simulink subsystem "mode_xxI"  (R2022a)
settings: Solver=VariableStepAuto  StartTime=0.0  StopTime=10.0  RelTol=1e-3
settings Model: Creator=bkfre  LastModifiedBy=bkfre

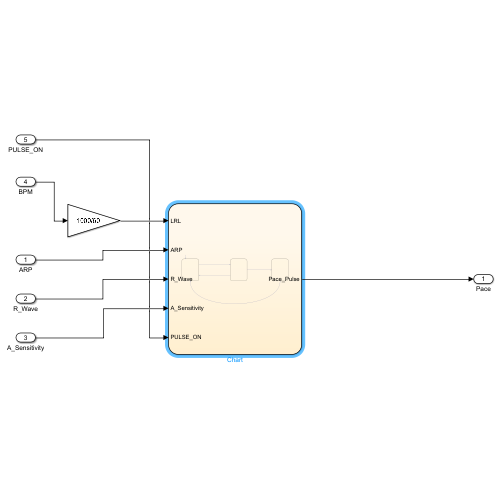
[thumbnail: Simulink's stored preview of the top-level diagram]
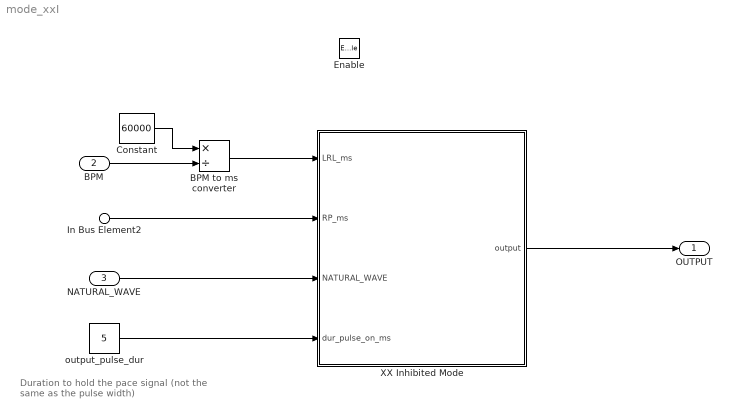
== system mode_xxI ==
  note: Duration to hold the pace signal (not the same as the pulse width)
  In Bus Element2 : Inport  PortName=BusSPECIFIC  Element=RP
  BPM : Inport  Port=2  OutDataTypeStr=double
  NATURAL_WAVE : Inport  Port=3
  Enable : EnablePort
  BPM to ms converter : Product  Inputs=*/
  Constant : Constant  Value=60000
  XX Inhibited Mode : Stateflow chart  TreatAsAtomicUnit=on
  output_pulse_dur : Constant  Value=5
  OUTPUT : Outport
  wires:
  Constant/1 -> BPM to ms converter/1
  NATURAL_WAVE/1 -> XX Inhibited Mode/3(NATURAL_WAVE)
  In Bus Element2/1 -> XX Inhibited Mode/2(RP_ms)
  output_pulse_dur/1 -> XX Inhibited Mode/4(dur_pulse_on_ms)
  BPM to ms converter/1 -> XX Inhibited Mode/1(LRL_ms)
  BPM/1 -> BPM to ms converter/2
  XX Inhibited Mode/1(output) -> OUTPUT/1

== stateflow chart mode_xxI/XX Inhibited Mode ==
  state Refractory
    entry:
    output=0;
  state Alert
  state Pace
    entry:
    output=1;
  note: If no natural wave detected before LRL interval expires, trigger an artificial pace
  note: If natural wave detected after refractory period, reset
  state Delay
    % keeps timing symmetrical whether
    % a natural wave or pacing occurs
  Pace -> Refractory : after(dur_pulse_on_ms,msec)
  (default) -> Refractory
  Refractory -> Alert : after(RP_ms-dur_pulse_on_ms,msec)
  Alert -> Pace [order 2] : after(LRL_ms-RP_ms,msec)
  Alert -> Delay [order 1] : [NATURAL_WAVE]
  Delay -> Refractory : after(dur_pulse_on_ms,msec)
  data: LRL_ms input; output output; RP_ms input; NATURAL_WAVE input; dur_pulse_on_ms input
